simulink library "nonentVNCApplied"  (R2022b)
settings: Solver=VariableStepAuto  StartTime=0.0  StopTime=10.0  RelTol=1e-3
undefined symbols (not defined in the file or in its folder): L
libraries: NonEntVncAppliedBtc x1
settings Model: Creator=ms51507  LastModifiedBy=kl13806
settings SolverCC: AlgebraicLoopSolver=TrustRegion
settings DebuggingCC: UnconnectedInputMsg=warning  UnconnectedOutputMsg=warning  UnconnectedLineMsg=warning  SFMachineParentedDataDiag=warning
settings ModelReferenceCC: EnableRefExpFcnMdlSchedulingChecks=on
settings RTWCC: DLArmComputeVersion=19.05

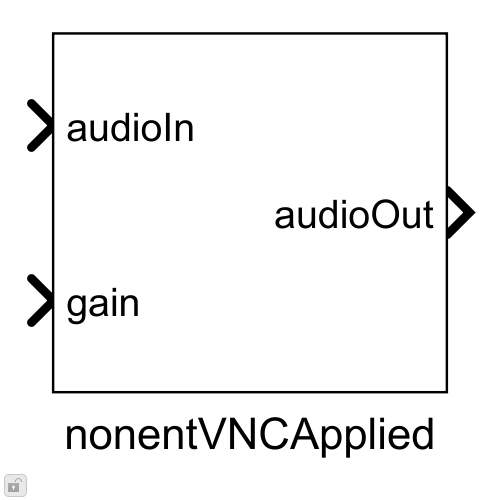
[thumbnail: Simulink's stored preview of the top-level diagram]
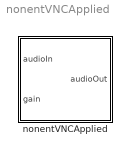
== system nonentVNCApplied ==
  nonentVNCApplied : Subsystem  mask(Bose nonentVNCApplied){L=L}
      mask prompts: L "FrameSize"
      mask init:
      | blkh = gcbh;
      | % Copy discrete mask parameters into a classdef object
      | InnerLinkConfig = NonEntVncAppliedConfig;
      | InnerLinkConfig.FrameSize = L;

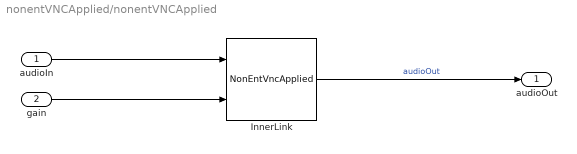
== system nonentVNCApplied/nonentVNCApplied ==
  audioIn : Inport
  gain : Inport  Port=2
  InnerLink : NonEntVncAppliedBtc/NonEntVncApplied  Config=InnerLinkConfig  FeatureName=VNC
      settings: SourceProductName=Bose Blocklib
  audioOut : Outport
  wires:
  InnerLink/1 -> audioOut/1  "audioOut"
  audioIn/1 -> InnerLink/1
  gain/1 -> InnerLink/2
